simulink model "diff_equastion"  (R2024a)
settings: Solver=VariableStepAuto  StartTime=0.0  StopTime=2  MaxStep=0.001  RelTol=1e-3
settings Model: Creator=xeon_ssd  LastModifiedBy=xeon_ssd

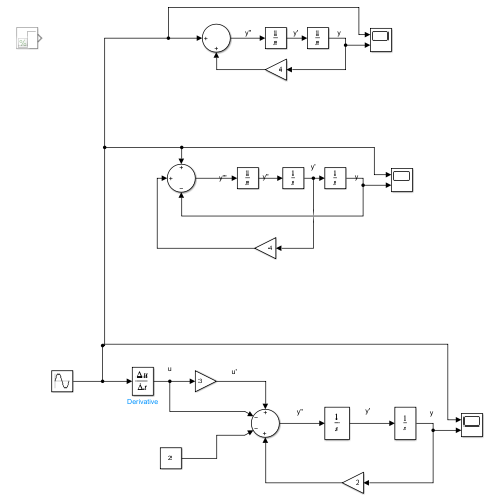
[thumbnail: Simulink's stored preview of the top-level diagram]
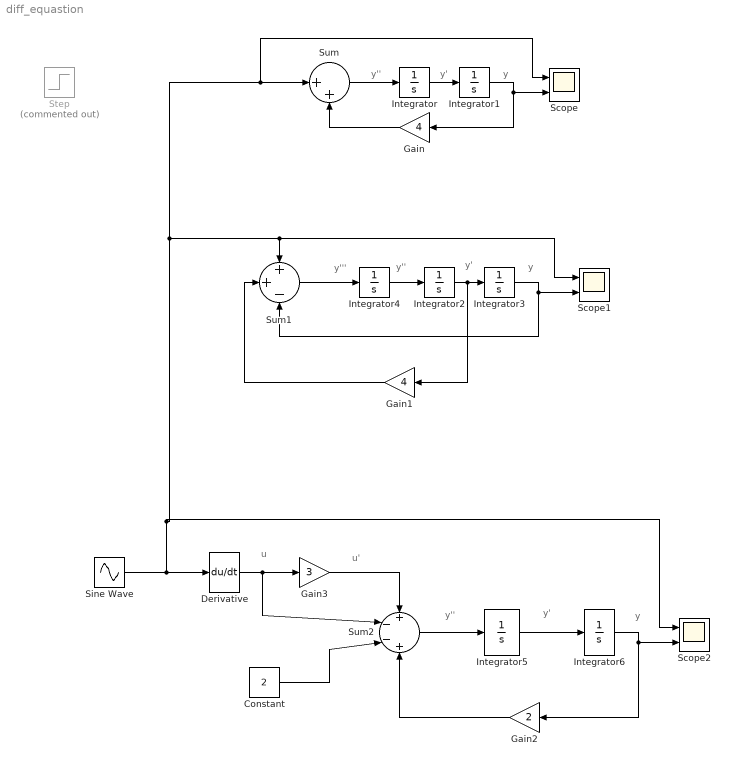
== system diff_equastion ==
  note: y
  note: y'
  note: y''
  note: u'
  note: u
  note: y'''
  note: y''
  note: y'
  note: y
  note: y''
  note: y'
  note: y
  Constant : Constant  Value=2
  Derivative : Derivative
  Gain : Gain  Gain=4
  Gain1 : Gain  Gain=4
  Gain2 : Gain  Gain=2
  Gain3 : Gain  Gain=3
  Integrator{,1..6} (7 alike) : Integrator
  Scope : Scope  NumInputPorts=2
  Scope1 : Scope  NumInputPorts=2
  Scope2 : Scope  NumInputPorts=2
  Sine Wave : Sin  Amplitude=10  Frequency=1*2*pi  SampleTime=0
  Step : Step  Commented=on  SampleTime=0
  Sum : Sum  Inputs=|++
  Sum1 : Sum  Inputs=++-
  Sum2 : Sum  Inputs=+--+
  wires:
  Sum/1 -> Integrator/1
  Integrator/1 -> Integrator1/1
  Integrator1/1 -> Scope/2, Gain/1
  Gain/1 -> Sum/2
  Integrator3/1 -> Sum1/3, Scope1/2
  Integrator2/1 -> Gain1/1, Integrator3/1
  Integrator4/1 -> Integrator2/1
  Sum1/1 -> Integrator4/1
  Gain1/1 -> Sum1/2
  Integrator5/1 -> Integrator6/1
  Sum2/1 -> Integrator5/1
  Integrator6/1 -> Scope2/2, Gain2/1
  Gain2/1 -> Sum2/4
  Derivative/1 -> Sum2/2, Gain3/1
  Gain3/1 -> Sum2/1
  Constant/1 -> Sum2/3
  Sine Wave/1 -> Scope/1, Sum/1, Scope1/1, Sum1/1, Scope2/1, Derivative/1
